simulink model "window_in_window_out_var_size"  (R2019b)
settings: Solver=VariableStepAuto  StartTime=0.0  StopTime=130  RelTol=1e-3
InitFcn:
  | xmcCheckSlxPath(bdroot)
  | load('data/input_1.txt')
undefined symbols (not defined in the file): xc7vx485tffg1157
libraries: ModelComposer x2, dspsrcs4 x1
settings Model: Creator=viswanad  LastModifiedBy=abehbood
settings SFSimCC: CustomCodeUndefinedFunction=UseInterfaceOnly

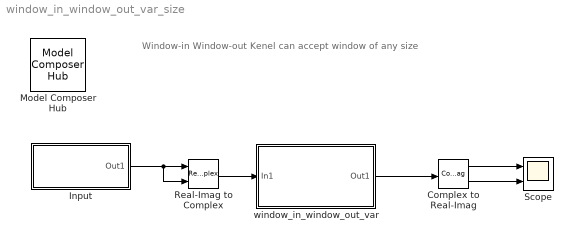
== system window_in_window_out_var_size ==
  note: Window-in Window-out
      | Kenel can accept window of any size
  Complex to Real-Imag : ComplexToRealImag
  Input : Subsystem
  Model Composer Hub : ModelComposer/Model Composer Hub  CodeGeneration=off  SubsystemName=window_in_window_out_var  TargetDirectory=./code  ExportType=AI Engines  IpVendor=xilinx.com  IpLibrary=hls  IpVersion=1.0  IpHWLanguage=Verilog  AieCompilerOptions={}  CreateTestbench=on  TestbenchStackSize=10  RunAieSim=on  AieSimTimeout=50000  LaunchVitisAnalyzer=off  RunX86Sim=on  X86SimTimeout=10  ProjDevice=xc7vx485tffg1157-1  ProjDevicePart=xc7vx485tffg1157-1  SamplePeriod=-1  ClockFrequency=200  DataPathParallelism=1
  Real-Imag to Complex : RealImagToComplex
  Scope : Scope  NumInputPorts=2
  window_in_window_out_var : Subsystem
  wires:
  Input/1(Out1) -> Real-Imag to Complex/2, Real-Imag to Complex/1
  window_in_window_out_var/1(Out1) -> Complex to Real-Imag/1
  Real-Imag to Complex/1 -> window_in_window_out_var/1(In1)
  Complex to Real-Imag/1 -> Scope/1
  Complex to Real-Imag/2 -> Scope/2

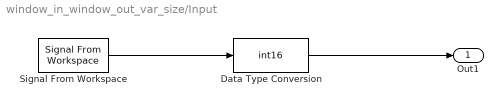
== system window_in_window_out_var_size/Input ==
  Data Type Conversion : DataTypeConversion  OutDataTypeStr=int16
  Signal From Workspace : dspsrcs4/Signal From Workspace  X=1:128  Ts=1  nsamps=20  OutputAfterFinalValue=Setting to zero  ignoreOrWarnInputAndFrameLengths=off  OutputFrames=off
  Out1 : Outport  VectorParamsAs1DForOutWhenUnconnected=off
  wires:
  Signal From Workspace/1 -> Data Type Conversion/1
  Data Type Conversion/1 -> Out1/1

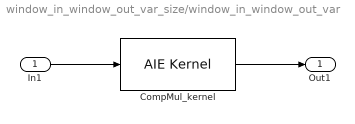
== system window_in_window_out_var_size/window_in_window_out_var ==
  In1 : Inport
  CompMul_kernel : ModelComposer/AIE Kernel  PortAttributesTable={ 'Input','in1','input_window_cint16 *','20','0','auto','';'Output','outw','output_window_cint16 *','20','','auto','' }  PortAttributesEnablement={'off', 'off', 'off', 'on', 'on', 'on', 'off';'off', 'off', 'off', 'on', 'off', 'on', 'off'}  FormalArgDecls={'input_window_cint16 * in1', 'output_window_cint16 * outw'}  PortWindowSizes={2.000000000000000000e+01, 2.000000000000000000e+01}  PortWindowMargins={0.000000000000000000e+00, 0.000000000000000000e+00}  PortSynchronicities={ 'auto','auto' }  PortSignalSizes={0.000000000000000000e+00, 0.000000000000000000e+00}  SimLibPath=''  FunctionTabVisible=on  FunctionDescription=void CompMul_kernel(input_window_cint16 * in1, output_window_cint16 * outw)  KernelHeaderFile=src/kernels/test_w2.h  KernelFunction=CompMul_kernel  KernelFunctionSelect=<empty>  KernelSourceFile=src/kernels/test_w2.cc  KernelSearchPaths={}  PreProcOptions={}  CoreRuntimeRatio=0.9
  Out1 : Outport  VectorParamsAs1DForOutWhenUnconnected=off
  wires:
  CompMul_kernel/1 -> Out1/1
  In1/1 -> CompMul_kernel/1
